simulink model "QPSK_Arm"  (R2016b)
settings: Solver=VariableStepAuto  StartTime=0.0  StopTime=10.0  RelTol=1e-3
libraries: commfilt2 x2, dspquant2 x2
settings Model: Creator=charles  LastModifiedBy=charles

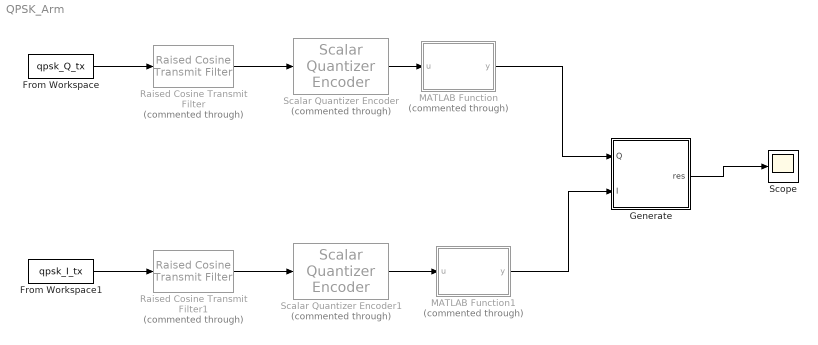
== system QPSK_Arm ==
  From Workspace : FromWorkspace  VariableName=qpsk_Q_tx  OutputAfterFinalValue=Holding final value
  From Workspace1 : FromWorkspace  VariableName=qpsk_I_tx  OutputAfterFinalValue=Holding final value
  "Generate " : MATLAB Function  TreatAsAtomicUnit=on
  MATLAB Function : MATLAB Function  Commented=through  TreatAsAtomicUnit=on
  MATLAB Function1 : MATLAB Function  Commented=through  TreatAsAtomicUnit=on
  Raised Cosine Transmit Filter : commfilt2/Raised Cosine Transmit Filter  Commented=through  filtType=Square root  R=0.2  filtSpan=10  N=8  filterGain=1  InputProcessing=Columns as channels (frame based)  RateOptions=Enforce single-rate processing  framing=Mute  checkCoeff=off  variableName=rcTxFilt  checkGain=Normalized  sampMode=Mute  saveAsFlag=0  currentFiltSpan=10  D=(10)/2  launchFVT=on  roundingMode=Floor  overflowMode=off  coeffDataTypeStr=Inherit: Same word length as input  coeffMin=[]  coeffMax=[]  coeffLastDataTypeStr=Inherit: Same word length as input  outputDataTypeStr=Inherit: Same as accumulator  outputMin=[]  outputMax=[]  outputLastDataTypeStr=Inherit: Same as accumulator
  Raised Cosine Transmit Filter1 : commfilt2/Raised Cosine Transmit Filter  Commented=through  filtType=Square root  R=0.2  filtSpan=10  N=8  filterGain=1  InputProcessing=Columns as channels (frame based)  RateOptions=Enforce single-rate processing  framing=Mute  checkCoeff=off  variableName=rcTxFilt1  checkGain=Normalized  sampMode=Mute  saveAsFlag=0  currentFiltSpan=10  D=(10)/2  launchFVT=on  roundingMode=Floor  overflowMode=off  coeffDataTypeStr=Inherit: Same word length as input  coeffMin=[]  coeffMax=[]  coeffLastDataTypeStr=Inherit: Same word length as input  outputDataTypeStr=Inherit: Same as accumulator  outputMin=[]  outputMax=[]  outputLastDataTypeStr=Inherit: Same as accumulator
  Scalar Quantizer Encoder : dspquant2/Scalar Quantizer Encoder  Commented=through  paramSrc=Specify via dialog  partType=Bounded  BBoundary=[1:10]  UBoundary=[2:9]  SearchMethod=Linear  tieBreakRule=Choose the lower index  outQU=off  outQError=off  codebook=[1.5:9.5]  outStatus=off  invalidin=Clip  idtype=int32  roundingMode=Floor  overflowMode=off
  Scalar Quantizer Encoder1 : dspquant2/Scalar Quantizer Encoder  Commented=through  paramSrc=Specify via dialog  partType=Bounded  BBoundary=[1:10]  UBoundary=[2:9]  SearchMethod=Linear  tieBreakRule=Choose the lower index  outQU=off  outQError=off  codebook=[1.5:9.5]  outStatus=off  invalidin=Clip  idtype=int32  roundingMode=Floor  overflowMode=off
  Scope : Scope
  wires:
  Raised Cosine Transmit Filter/1 -> Scalar Quantizer Encoder/1
  Scalar Quantizer Encoder/1 -> MATLAB Function/1(u)
  Raised Cosine Transmit Filter1/1 -> Scalar Quantizer Encoder1/1
  Scalar Quantizer Encoder1/1 -> MATLAB Function1/1(u)
  From Workspace/1 -> Raised Cosine Transmit Filter/1
  From Workspace1/1 -> Raised Cosine Transmit Filter1/1
  MATLAB Function/1(y) -> "Generate "/1(Q)
  MATLAB Function1/1(y) -> "Generate "/2(I)
  "Generate "/1(res) -> Scope/1

== matlab function QPSK_Arm/MATLAB Function1 ==
  data: u input; y output
function y = fcn(u)

y = u;

== matlab function QPSK_Arm/MATLAB Function ==
  data: u input; y output
function y = fcn(u)

y = u;

== matlab function QPSK_Arm/Generate  ==
  data: Q input; I input; res output
function res  = fcn(Q, I)
%-------------Generation du signal QPSK
%%%%%%%%%%%%%%%%%%% Variables à utiliser %%%%%%%%%%%%%%%%%%%%%

nsb = 30		%Nombre de bits

fb = 1e5		%Fréquence des bits
Tb = 1/fb		%Période des bits
Eb = 1			%Energie par bit
T = 2*Tb		%Période des symboles
Nsymb = nsb/2   %Nombre de symboles

fc = 1e6		%Fréquence de la porteuse (carrier)

Ts = 1/(10*fc)	%Période d'échantillonnage : définit le pas de simulation
fs = 1/Ts		%Fréquence d'échantillonnage

npb = round(Tb/Ts)		%Nombre de points par bit

t = [Ts:Ts:nsb*Tb];     %Vecteur représentant l'axe du temps
I=I(:).';
Q=Q(:).';
res = 2*sqrt(Eb/T).* cos(2*pi*fc.*t - Q.*(pi/2 - I*pi/4));
